simulink model "PODPWM"  (R2021b)
settings: Solver=ode45  StartTime=0.0  StopTime=0.5  MaxStep=1e-6  RelTol=1e-5
libraries: spsMosfetLib x8, simulink x4, spsVoltageMeasurementLib x3, spsDCVoltageSourceLib x2, spsSeriesRLCBranchLib x1, spspowerguiLib x1
settings Model: Creator=singh  LastModifiedBy=singh
settings DataIOCC: ReturnWorkspaceOutputs=off

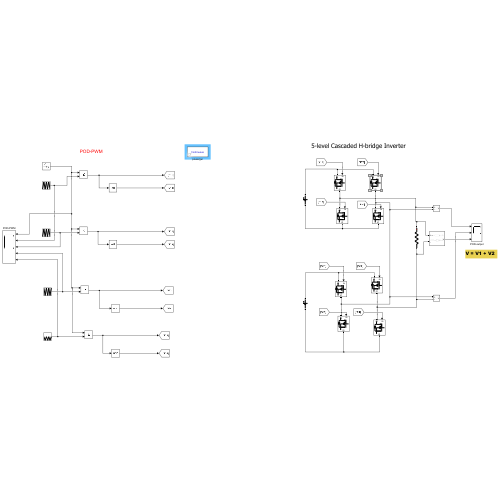
[thumbnail: Simulink's stored preview of the top-level diagram]
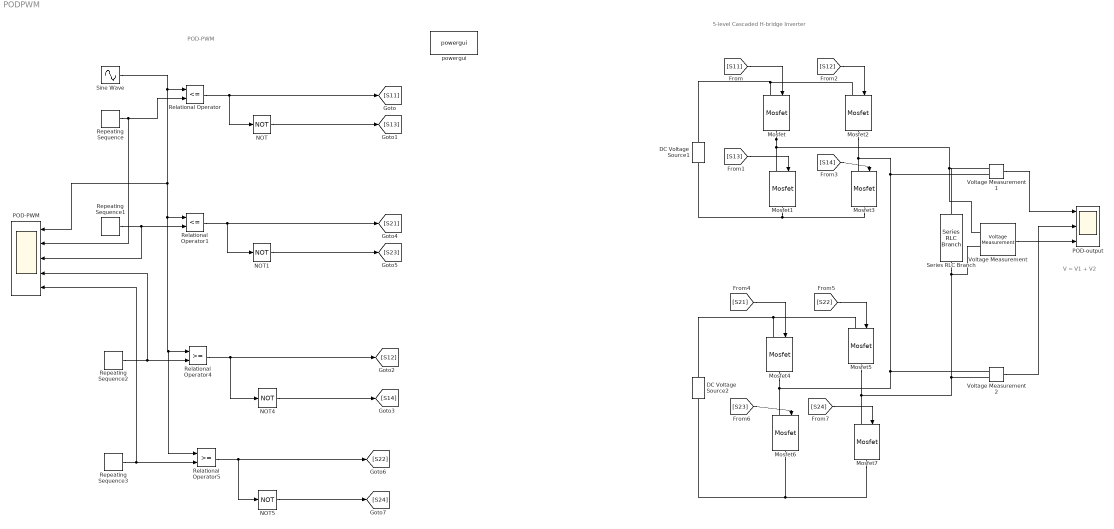
== system PODPWM ==
  note: V = V1 + V2
  note: POD-PWM
  note: 5-level Cascaded H-bridge Inverter
  DC Voltage Source1 : spsDCVoltageSourceLib/DC Voltage Source  Amplitude=100  Measurements=None
  DC Voltage Source2 : spsDCVoltageSourceLib/DC Voltage Source  Amplitude=100  Measurements=None
  Mosfet{,1..7} (8 alike) : spsMosfetLib/Mosfet  Ron=0.1  Lon=0  Rd=0.01  Vfd=0  IC=0  Rs=1e5  Cs=inf  Measurements=off
  NOT{,1,4..5} (4 alike) : Logic  Operator=NOT  AllPortsSameDT=off  OutDataTypeStr=boolean
  POD-PWM : Scope  NumInputPorts=5
  POD-output : Scope  NumInputPorts=3
  Relational Operator : RelationalOperator  Operator=<=  OutDataTypeStr=boolean  RndMeth=Simplest
  Relational Operator1 : RelationalOperator  Operator=<=  OutDataTypeStr=boolean  RndMeth=Simplest
  Relational Operator4 : RelationalOperator  OutDataTypeStr=boolean  RndMeth=Simplest
  Relational Operator5 : RelationalOperator  OutDataTypeStr=boolean  RndMeth=Simplest
  Repeating Sequence : simulink/Sources/Repeating Sequence  rep_seq_t=[0 0.5 1]*1/10000  rep_seq_y=[0 1 0]
  Repeating Sequence1 : simulink/Sources/Repeating Sequence  rep_seq_t=[0 0.5 1]*1/10000  rep_seq_y=[1 2 1]
  Repeating Sequence2 : simulink/Sources/Repeating Sequence  rep_seq_t=[0 0.5 1]*1/10000  rep_seq_y=[0 -1 0]
  Repeating Sequence3 : simulink/Sources/Repeating Sequence  rep_seq_t=[0 0.5 1]*1/10000  rep_seq_y=[-1 -2 -1]
  Series RLC Branch : spsSeriesRLCBranchLib/Series RLC Branch  LConnTagsString=__new0  RConnTagsString=__new0  BranchType=R  Resistance=100  Inductance=1e-3  SetiL0=off  InitialCurrent=0  Capacitance=1e-6  Setx0=off  InitialVoltage=0  Measurements=None
  Sine Wave : Sin  Amplitude=1.7  Frequency=50*2*pi  SampleTime=0
  Voltage Measurement : spsVoltageMeasurementLib/Voltage Measurement  PhasorSimulation=off  OutputType=Complex  PSBequivalent=0
  Voltage Measurement1 : spsVoltageMeasurementLib/Voltage Measurement  PhasorSimulation=off  OutputType=Complex  PSBequivalent=0
  Voltage Measurement2 : spsVoltageMeasurementLib/Voltage Measurement  PhasorSimulation=off  OutputType=Complex  PSBequivalent=0
  powergui : spspowerguiLib/powergui  Priority=1  SimulationMode=Continuous  SampleTime=50e-6  frequency=60  Iterations=50  frequencyindice=0  Pbase=100e6  ErrMax=1e-4  UnitsV=kV  UnitsW=MW  buscounter=0  FunctionMessages=off  echomessages=off  EnableUseOfTLC=off  CurrentSourceSwitches=off  DisableSnubberDevices=off  DisableRonSwitches=off  DisableVfSwitches=off  DisplayEquations=off  AutomaticDiscreteSolvers=off  SolverType=Tustin/Backward Euler (TBE)  Interpol=off  ExternalGateDelay=off  methode=off  Ts=100  x0status=blocks  SPID=on  SwTol=0  HookPort=off  NonlinearTolerance=1e-4  nMaxIteration=100  ContinueOnMaxIteration=off  RestoreLinks=warning  ResistiveCurrentMeasurement=off  Frange=[0:2:500]  Ylog=off  Xlog=on  ShowGrid=off  save=off  variable=ZData  structure=0  ZoomFFT=off  StartTime=0.0  cycles=1  DisplayStyle=1  fundamental=60  FreqAxis=off  MaxFrequency=1000  frequencyindicesteady=1  RmsSteady=1  display=off
  wires:
  Voltage Measurement1/1 -> POD-output/1
  Relational Operator/1 -> NOT/1, [S11]
  Voltage Measurement2/1 -> POD-output/2
  Relational Operator4/1 -> [S12], NOT4/1
  Relational Operator1/1 -> NOT1/1, [S21]
  Repeating Sequence2/1 -> Relational Operator4/2, POD-PWM/4
  NOT1/1 -> [S23]
  [S21] -> Mosfet4/1
  Repeating Sequence1/1 -> POD-PWM/3, Relational Operator1/2
  Repeating Sequence3/1 -> Relational Operator5/2, POD-PWM/5
  Voltage Measurement/1 -> POD-output/3
  NOT4/1 -> [S14]
  [S12] -> Mosfet2/1
  [S14] -> Mosfet3/1
  [S24] -> Mosfet7/1
  [S11] -> Mosfet/1
  NOT/1 -> [S13]
  Sine Wave/1 -> POD-PWM/1, Relational Operator5/1, Relational Operator4/1, Relational Operator1/1, Relational Operator/1
  [S22] -> Mosfet5/1
  [S23] -> Mosfet6/1
  NOT5/1 -> [S24]
  [S13] -> Mosfet1/1
  Relational Operator5/1 -> [S22], NOT5/1
  Repeating Sequence/1 -> POD-PWM/2, Relational Operator/2
  connections:
  Mosfet5/RConn1 -- Mosfet7/LConn1 -- Series RLC Branch/RConn1 -- Voltage Measurement/LConn2 -- Voltage Measurement2/LConn2
  Mosfet4/LConn1 -- Mosfet5/LConn1 -- DC Voltage Source2/RConn1
  Mosfet/LConn1 -- Mosfet2/LConn1 -- DC Voltage Source1/RConn1
  Mosfet2/RConn1 -- Mosfet3/LConn1 -- Voltage Measurement1/LConn2 -- Mosfet6/LConn1 -- Mosfet4/RConn1 -- Voltage Measurement2/LConn1
  Mosfet6/RConn1 -- DC Voltage Source2/LConn1 -- Mosfet7/RConn1
  Mosfet1/RConn1 -- Mosfet3/RConn1 -- DC Voltage Source1/LConn1
  Mosfet/RConn1 -- Mosfet1/LConn1 -- Series RLC Branch/LConn1 -- Voltage Measurement/LConn1 -- Voltage Measurement1/LConn1
